simulink model "system_main"  (R2023b)
settings: Solver=VariableStepAuto  StartTime=0.0  StopTime=10.0  RelTol=1e-3
settings Model: Creator=gio  LastModifiedBy=gio

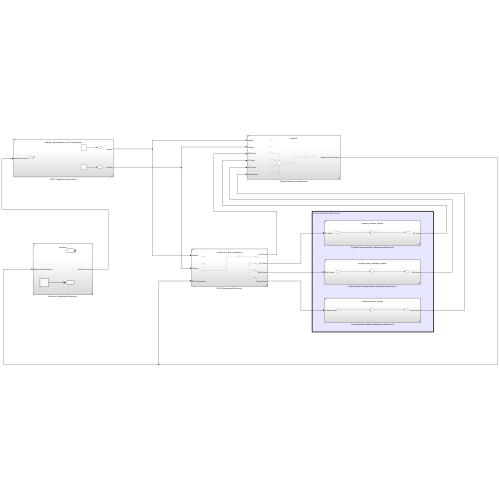
[thumbnail: Simulink's stored preview of the top-level diagram]
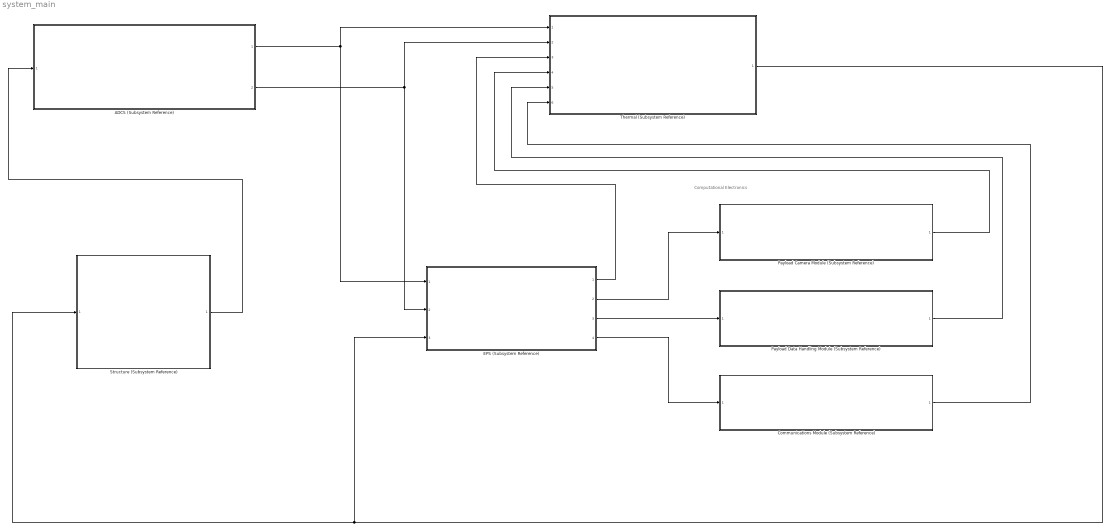
== system system_main ==
  note: Computational Electronics
  ADCS (Subsystem Reference) : Subsystem  ReferencedSubsystem=attitude_determination_control_subsystem
  Communications Module (Subsystem Reference) : Subsystem  ReferencedSubsystem=communications_module
  EPS (Subsystem Reference) : Subsystem  ReferencedSubsystem=electrical_power_subsystem
  Payload Camera Module (Subsystem Reference) : Subsystem  ReferencedSubsystem=payload_camera_module
  Payload Data Handling Module (Subsystem Reference) : Subsystem  ReferencedSubsystem=payload_data_handling_module
  Structure (Subsystem Reference) : Subsystem  ReferencedSubsystem=structure
  Thermal (Subsystem Reference) : Subsystem  ReferencedSubsystem=thermal
  wires:
  EPS (Subsystem Reference)/2 -> Payload Camera Module (Subsystem Reference)/1
  EPS (Subsystem Reference)/3 -> Payload Data Handling Module (Subsystem Reference)/1
  EPS (Subsystem Reference)/4 -> Communications Module (Subsystem Reference)/1
  Communications Module (Subsystem Reference)/1 -> Thermal (Subsystem Reference)/6
  Payload Data Handling Module (Subsystem Reference)/1 -> Thermal (Subsystem Reference)/5
  Payload Camera Module (Subsystem Reference)/1 -> Thermal (Subsystem Reference)/4
  EPS (Subsystem Reference)/1 -> Thermal (Subsystem Reference)/3
  Thermal (Subsystem Reference)/1 -> Structure (Subsystem Reference)/1, EPS (Subsystem Reference)/3
  ADCS (Subsystem Reference)/1 -> Thermal (Subsystem Reference)/1, EPS (Subsystem Reference)/1
  ADCS (Subsystem Reference)/2 -> Thermal (Subsystem Reference)/2, EPS (Subsystem Reference)/2
  Structure (Subsystem Reference)/1 -> ADCS (Subsystem Reference)/1
